simulink model "lab_6_simulink"  (R2024b)
settings: Solver=ode45  StartTime=0.0  StopTime=50.0  MaxStep=1/32  RelTol=1e-3
libraries: simulink x2
settings Model: Creator=lw53894  LastModifiedBy=lw53894

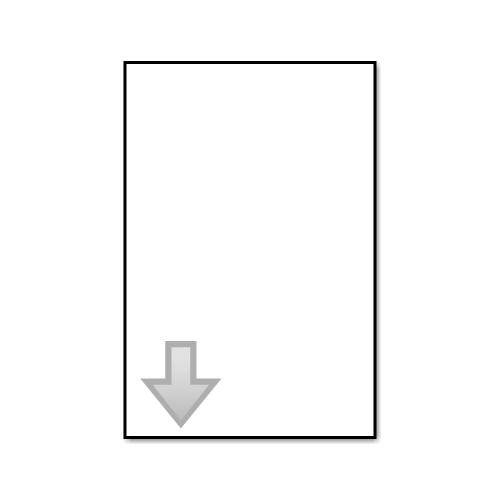
[thumbnail: Simulink's stored preview of the top-level diagram]
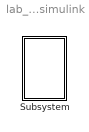
== system lab_6_simulink ==
  Subsystem : Subsystem  mask{g=9.81, m1=0.5, m2=0.9, M=1, R=0.001, r0=1, theta0=120}

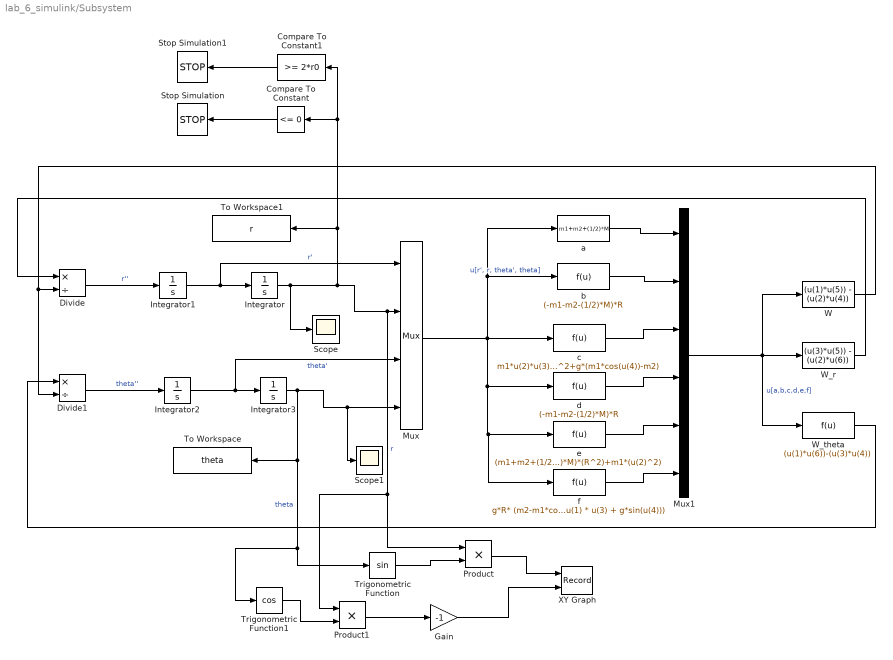
== system lab_6_simulink/Subsystem ==
  Compare To Constant : simulink/Logic and Bit Operations/Compare To Constant  relop=<=  const=0  OutDataTypeStr=boolean
  Compare To Constant1 : simulink/Logic and Bit Operations/Compare To Constant  relop=>=  const=2*r0  OutDataTypeStr=boolean
  Divide : Product  Inputs=*/
  Divide1 : Product  Inputs=*/
  Gain : Gain  Gain=-1
  Integrator : Integrator  InitialCondition=r0
  Integrator1 : Integrator
  Integrator2 : Integrator
  Integrator3 : Integrator  InitialCondition=(theta0*pi)/180
  Mux : Mux
  Mux1 : Mux  Inputs=6
  Product : Product
  Product1 : Product
  Scope : Scope
  Scope1 : Scope
  Stop Simulation : Stop
  Stop Simulation1 : Stop
  To Workspace : ToWorkspace  VariableName=theta  SaveFormat=Timeseries  SampleTime=-1
  To Workspace1 : ToWorkspace  VariableName=r  SaveFormat=Timeseries  SampleTime=-1
  Trigonometric Function : Trigonometry
  Trigonometric Function1 : Trigonometry  Operator=cos
  W : Fcn  Expr=(u(1)*u(5)) - (u(2)*u(4))
  W_r : Fcn  Expr=(u(3)*u(5)) - (u(2)*u(6))
  W_theta : Fcn  Expr=(u(1)*u(6))-(u(3)*u(4))
  XY Graph : Record  FileSettingsInternal="{\"entries\":[{\"content\":{\"excelSettings\":{\"content\":{},\"type\":\"Streamout.ExcelSettings\"}},\"type\":\"Streamout.FileSettingStorage\",\"uuid\":\"\"}],\"packageUris\":[\"http:\\/\\/schema.mathworks.com\\/mf0\\/streamout_blocks\\/R2020a\"],\"version\":\"1.0\"}"  Layout=[1 1]  SignalsInternal="{\"entries\":[{\"content\":{\"signals\":[{\"content\":{\"blockPath\":[],\"dimensions\":[1],\"domain\":\"\",\"lineColor\":\"#a2142f\",\"plots\":[ 1 ],\"port\":1,\"sid\":[\"\"],\"signalID\":1,\"signalName\":\"Product\"},\"type\":\"RecordBlkView.Signal\",\"uuid\":\"\"},{\"content\":{\"blockPath\":[],\"dimensions\":[1],\"domain\":\"\",\"lineColor\":\"#139fff\",\"plots\":[ 1 ],\"port\":2,\"sid\":[\"\"],\"signalID\":2,\"signalName\":\"Gain\"},\"type\":\"RecordBlkView.Signal\",\"uuid\":\"\"}]},\"type\":\"RecordBlkView.InputSignals\",\"uuid\":\"\"}],\"packageUris\":[\"http:\\/\\/schema.mathworks.com\\/mf0\\/streamout_blocks\\/R2020a\"],\"version\":\"1.0\"}"  VisualizationBindings="{\"xyplotplugin\":{\"info\":[{\"series\":[{\"bindingParametersList\":[{\"parameter\":\"X-Axis\",\"signalID\":1,\"signalName\":\"Product\"},{\"parameter\":\"Y-Axis\",\"signalID\":2,\"signalName\":\"Gain\"}],\"seriesID\":0}],\"subplotID\":1}]}}"  CompatibilityTag=XY
  a : Fcn  Expr=m1+m2+(1/2)*M
  b : Fcn  Expr=(-m1-m2-(1/2)*M)*R
  c : Fcn  Expr=m1*u(2)*u(3)^2+g*(m1*cos(u(4))-m2)
  d : Fcn  Expr=(-m1-m2-(1/2)*M)*R
  e : Fcn  Expr=(m1+m2+(1/2)*M)*(R^2)+m1*(u(2)^2)
  f : Fcn  Expr=g*R* (m2-m1*cos(u(4))) - m1*u(2) * (2*u(1) * u(3) + g*sin(u(4)))
  wires:
  b/1 -> Mux1/2
  d/1 -> Mux1/4
  W_r/1 -> Divide/1
  Mux/1 -> c/1, b/1, a/1, f/1, e/1, d/1  "u[r', r, theta', theta]"
  Mux1/1 -> W_theta/1, W/1, W_r/1  "u[a,b,c,d,e,f]"
  f/1 -> Mux1/6
  a/1 -> Mux1/1
  Integrator2/1 -> Mux/3, Integrator3/1  "theta'"
  c/1 -> Mux1/3
  e/1 -> Mux1/5
  Integrator1/1 -> Mux/1, Integrator/1  "r'"
  Divide/1 -> Integrator1/1  "r''"
  W_theta/1 -> Divide1/1
  Integrator3/1 -> To Workspace/1, Trigonometric Function1/1, Trigonometric Function/1, Scope1/1, Mux/4  "theta"
  Integrator/1 -> Scope/1, To Workspace1/1, Compare To Constant1/1, Compare To Constant/1, Product1/1, Product/1, Mux/2  "r"
  W/1 -> Divide1/2, Divide/2
  Divide1/1 -> Integrator2/1  "theta''"
  Trigonometric Function/1 -> Product/2
  Product/1 -> XY Graph/1
  Trigonometric Function1/1 -> Product1/2
  Product1/1 -> Gain/1
  Gain/1 -> XY Graph/2
  Compare To Constant/1 -> Stop Simulation/1
  Compare To Constant1/1 -> Stop Simulation1/1
